simulink model "modelforpresentation"  (R2022a)
settings: Solver=ode45  StartTime=0.0  StopTime=1.7  RelTol=1e-3
undefined symbols (not defined in the file): vehicle_speed, wheel_speed
settings Model: Creator=Dell  LastModifiedBy=prabhi

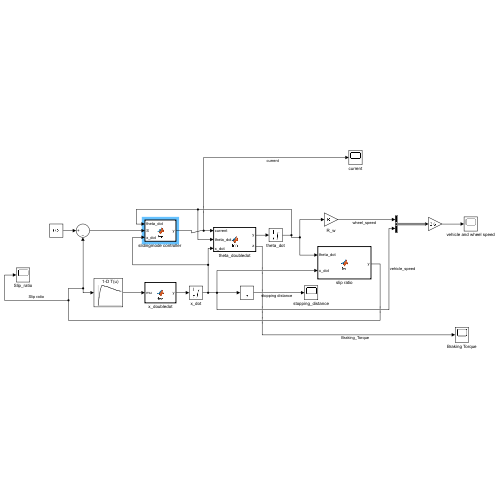
[thumbnail: Simulink's stored preview of the top-level diagram]
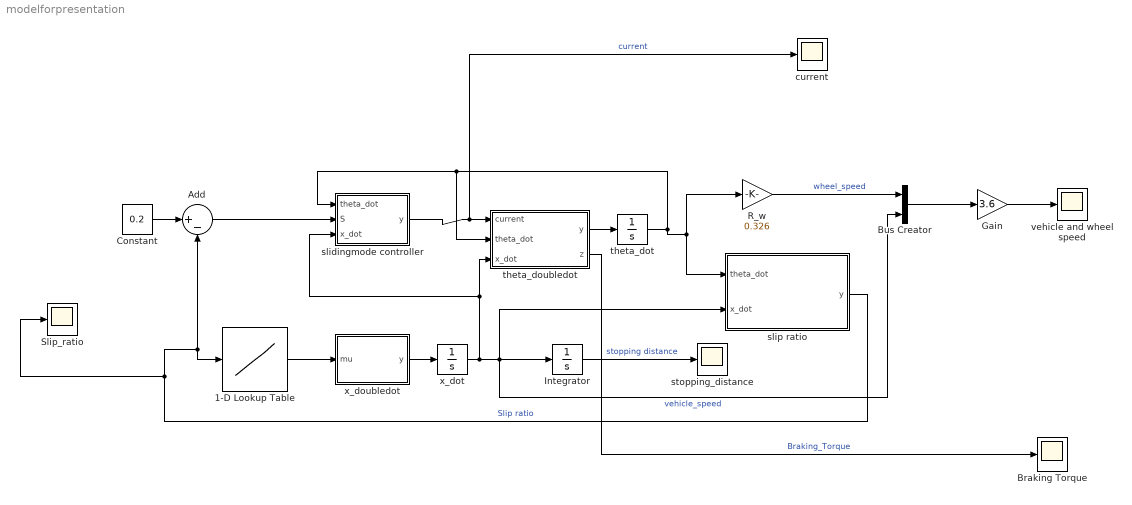
== system modelforpresentation ==
  1-D Lookup Table : Lookup_n-D  NumberOfTableDimensions=1  BreakpointsForDimension1=|  Table=|  InterpMethod=Linear Lagrange  InternalRulePriority=Speed  RndMeth=Simplest
      BreakpointsForDimension1=|
      | [0
      | 0.0500000000000000028
      | 0.100000000000000006
      | 0.150000000000000022
      | 0.200000000000000011
      | 0.25
      | 0.300000000000000044
      | 0.350000000000000033
      | 0.400000000000000022
      | 0.450000000000000011
      | 0.5
      | 0.550000000000000044
      | 0.599999999999999978
      | 0.649999999999999911
      | 0.699999999999999956
      | 0.75
      | 0.800000000000000044
      | 0.849999999999999978
      | 0.900000000000000022
      | 0.949999999999999956
      | 1]
      Table=|
      | [0
      | 0.400000000000000022
      | 0.800000000000000044
      | 0.969999999999999973
      | 1
      | 0.979999999999999982
      | 0.959999999999999964
      | 0.939999999999999947
      | 0.92000000000000004
      | 0.900000000000000022
      | 0.880000000000000004
      | 0.854999999999999982
      | 0.82999999999999996
      | 0.810000000000000053
      | 0.790000000000000036
      | 0.770000000000000018
      | 0.75
      | 0.729999999999999982
      | 0.719999999999999973
      | 0.709999999999999964
      | 0.699999999999999956]
  Add : Sum  Inputs=|+-
  Braking Torque : Scope
  Bus Creator : BusCreator  Inputs=wheel_speed,vehicle_speed
  Constant : Constant  Value=0.2
  Gain : Gain  Gain=3.6
  Integrator : Integrator
  R_w : Gain  Gain=0.326
  Slip_ratio : Scope
  current : Scope
  "slidingmode controller " : MATLAB Function  TreatAsAtomicUnit=on
  slip ratio : MATLAB Function  TreatAsAtomicUnit=on
  stopping_distance : Scope
  theta_dot : Integrator  InitialCondition=59.6455351  LimitOutput=on  UpperSaturationLimit=60  LowerSaturationLimit=0
  theta_doubledot : MATLAB Function  TreatAsAtomicUnit=on
  vehicle and wheel speed : Scope
  x_dot : Integrator  InitialCondition=19.444444  LimitOutput=on  UpperSaturationLimit=1000  LowerSaturationLimit=0
  x_doubledot : MATLAB Function  TreatAsAtomicUnit=on
  wires:
  Constant/1 -> Add/1
  Add/1 -> "slidingmode controller "/2(S)
  "slidingmode controller "/1(y) -> current/1, theta_doubledot/1(current)  "current"
  theta_doubledot/1(y) -> theta_dot/1
  slip ratio/1(y) -> Slip_ratio/1, 1-D Lookup Table/1, Add/2  "Slip ratio"
  x_doubledot/1(y) -> x_dot/1
  x_dot/1 -> slip ratio/2(x_dot), Bus Creator/2, Integrator/1, "slidingmode controller "/3(x_dot), theta_doubledot/3(x_dot)  "vehicle_speed"
  Integrator/1 -> stopping_distance/1  "stopping distance"
  Bus Creator/1 -> Gain/1
  R_w/1 -> Bus Creator/1  "wheel_speed"
  1-D Lookup Table/1 -> x_doubledot/1(mu)
  theta_dot/1 -> "slidingmode controller "/1(theta_dot), theta_doubledot/2(theta_dot), R_w/1, slip ratio/1(theta_dot)
  theta_doubledot/2(z) -> Braking Torque/1  "Braking_Torque"
  Gain/1 -> vehicle and wheel speed/1

== matlab function modelforpresentation/theta_doubledot ==
  data: current input; y output; theta_dot input; x_dot input; z output
function [y,z]= fcn(current, theta_dot,x_dot)
mu = 0.8 ;
g = 9.80665 ;
N = 4 ;
r_z = 0.168  ;
r_w = 0.118  ;
mu_p = 0.09 ;
h = 10^(-3) ;
k = 0.269 ;
alpha = 12.5 * 1000 ; 
I_y = 2.5 * 10^(-2)  ;
R_w = 0.326 ;
l = 2.5 ;
h_CE = 0.5 ;
m_w = 40 ;
m_v = 1630 ; 
I_t = 1.75 ;
f_0 = 10^ (-2) ;
f_s = 5*10^(-3) ;
K_v = 2.237 ;
T_i = 2*( pi )*N*k*alpha*(r_z^3 - r_w^3)/3 ; 
T_v = pi*N*mu_p*(r_z^4 - r_w^4) / (2*h) ;
m_t = 0.25*m_v + m_w ;
I = I_t + I_y ;
m_1 = m_v*h_CE/ (l*m_t) ;
x_doubledot = -mu*g/ (1+mu*m_1) ;
F_n = m_t*g - (m_v*h_CE*x_doubledot)/l ; 
t_i = T_i/I ;
t_v = T_v/I ;
t_n = R_w*F_n/I ;
F_r = f_0 + f_s*3.24*(K_v*x_dot)^(2.5) ;%input needed  
t_r = R_w*F_r/I ;
u = -t_i*current - t_v*theta_dot + mu*t_n- t_r ; 
T_b = T_i*current + T_v*theta_dot ;
z = T_b ;
y = u;

== matlab function modelforpresentation/slidingmode controller  ==
  data: theta_dot input; y output; S input; x_dot input
function y = fcn(theta_dot , S ,x_dot ) 
mu = 0.8 ;
s_rd = 0.2;
lambda = 5;
neeta  = 1.1 ;
g = 9.80665;
mu_star = 0.3;
N = 4 ;
r_z = 0.168  ;
r_w = 0.118  ;
mu_p = 0.09;
h = 10^(-3);
k = 0.269 ;
alpha = 12.5 * 1000 ;
I_y = 2.5 * 10^(-2)  ;

R_w = 0.326 ;
l = 2.5 ;
h_CE = 0.5 ;
m_w = 40 ;
m_v = 1630 ; 
I_t = 1.75 ;
f_0 = 10^ (-2) ;
f_s = 5*10^(-3) ;
K_v = 2.237 ;
T_i = 2*( pi )*N*k*alpha*(r_z^3 - r_w^3)/3 ; 
T_v = pi*N*mu_p*(r_z^4 - r_w^4) / (2*h) ;
m_t = 0.25*m_v + m_w ;
I = I_t + I_y ;
m_1 = m_v*h_CE/ (l*m_t) ;
x_doubledot = -mu*g/ (1+mu*m_1) ;
F_n = m_t*g - (m_v*h_CE*x_doubledot)/l ;
t_i = T_i/I ;
t_v = T_v/I ;
t_n = R_w*F_n/I ;
F_r = f_0 + f_s*3.24*(K_v*x_dot)^(2.5) ; %input needed  
t_r = R_w*F_r/I ; 
if abs(S) < 0.05 ; 
    sat = S/0.05 ;
else sat = sign(S) ;
end 
if (theta_dot ~= 0 ) & (x_dot ~= 0)
 u = mu*g*theta_dot/((1+mu*m_1)*x_dot*t_i) + (mu*t_n -t_r-t_v*theta_dot)/t_i+ lambda*theta_dot/t_i + x_dot*lambda*(s_rd-1)/(R_w*t_i)+ (neeta + mu_star*(g*theta_dot+x_dot*t_n)/x_dot)*sat/t_i ;
else u = 0 ; 
end
y = u;

== matlab function modelforpresentation/x_doubledot ==
  data: mu input; y output
function y = fcn(mu)
mu = 0.8 ;
s_rd = 0.2;
lambda = 5;
neeta  = 1.1 ;
g = 9.80665;
mu_star = 0.3;
N = 4 ;
r_z = 0.168  ;
r_w = 0.118  ;
mu_p = 0.09;
h = 10^(-3);
k = 0.269 ;
alpha = 12.5 * 1000 ;
I_y = 2.5 * 10^(-2)  ;

R_w = 0.326 ;
l = 2.5 ;
h_CE = 0.5 ;
m_w = 40 ;
m_v = 1630 ; 
I_t = 1.75 ;
f_0 = 10^ (-2) ;
f_s = 5*10^(-3) ;
K_v = 2.237 
g = 9.80665 ;
l = 2.5 ;
h_CE = 0.5 ;
m_w = 40 ;
m_v = 1630 ; 

m_t = 0.25*m_v + m_w ;

m_1 = m_v*h_CE/ (l*m_t) ;
x_doubledot = -mu*g/ (1+mu*m_1) ;

u = x_doubledot ;
y = u;

== matlab function modelforpresentation/slip ratio ==
  data: theta_dot input; x_dot input; y output
function y = fcn(theta_dot , x_dot)
R_w = 0.326;
mu = 0.8 ;
s_rd = 0.2;
lambda = 5;
neeta  = 1.1 ;
g = 9.80665;
mu_star = 0.3;
N = 4 ;
r_z = 0.168  ;
r_w = 0.118  ;
mu_p = 0.09;
h = 10^(-3);
k = 0.269 ;
alpha = 12.5 * 1000 ;
I_y = 2.5 * 10^(-2)  ;

R_w = 0.326 ;
l = 2.5 ;
h_CE = 0.5 ;
m_w = 40 ;
m_v = 1630 ; 
I_t = 1.75 ;
f_0 = 10^ (-2) ;
f_s = 5*10^(-3) ;
K_v = 2.237 
s_rd = (x_dot - R_w*theta_dot)/ x_dot
y = s_rd;
